simulink model "motor_control"  (R2023b)
settings: Solver=VariableStepAuto  StartTime=0.0  StopTime=3  RelTol=1e-3
model workspace (MAT data in the model file):
  K = 2.2
  Kp = 1
  Sig = Simulink.Signal
  Sig.DataType = 'auto'
  Sig.Dimensions = -1
  Sig.DimensionsMode = 'auto'
  Sig.Complexity = 'auto'
  Sig.SampleTime = -1
  Sig.SamplingMode = 'auto'
  sigma = 14
settings Model: Creator=realf  LastModifiedBy=realf

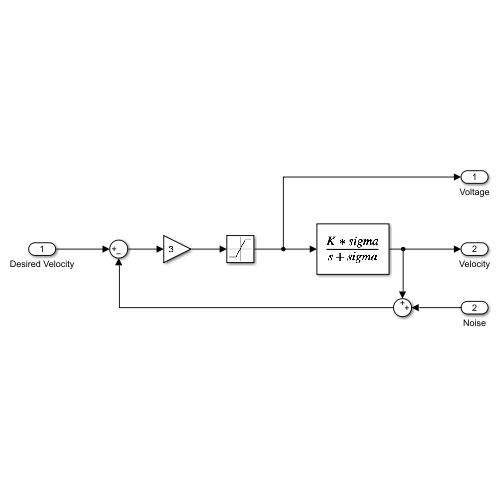
[thumbnail: Simulink's stored preview of the top-level diagram]
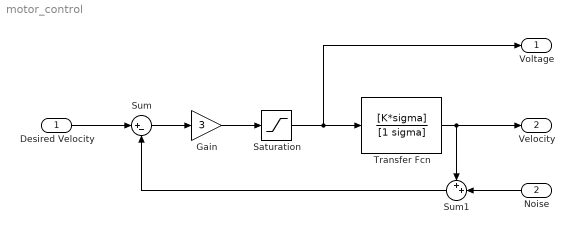
== system motor_control ==
  Desired Velocity : Inport
  Noise : Inport  Port=2
  Gain : Gain  Gain=3
  Saturation : Saturate  UpperLimit=7.5  LowerLimit=-7.5
  Sum : Sum  Inputs=|+-
  Sum1 : Sum  Inputs=++|
  Transfer Fcn : TransferFcn  Numerator=[K*sigma]  Denominator=[1 sigma]
  Voltage : Outport
  Velocity : Outport  Port=2
  wires:
  Desired Velocity/1 -> Sum/1
  Gain/1 -> Saturation/1
  Saturation/1 -> Voltage/1, Transfer Fcn/1
  Transfer Fcn/1 -> Velocity/1, Sum1/1
  Noise/1 -> Sum1/2
  Sum1/1 -> Sum/2
  Sum/1 -> Gain/1
